simulink model "GenericTargetTemplate"  (R2022b)
settings: Solver=FixedStepAuto  StartTime=0.0  StopTime=10.0  FixedStep=0.01  RelTol=1e-3  EnableMultiTasking=on
libraries: GenericTarget x3
settings Model: Creator=damerius  LastModifiedBy=damerius
settings SolverCC: ConcurrentTasks=on  AlgebraicLoopSolver=TrustRegion  PositivePriorityOrder=on
settings DataIOCC: SaveOutput=off  SignalLogging=off  DSMLogging=off  SaveTime=off  ReturnWorkspaceOutputs=off
settings OptimizationCC: DefaultParameterBehavior=Inlined  ZeroExternalMemoryAtStartup=off  ZeroInternalMemoryAtStartup=off  SimCompilerOptimization=on
settings DebuggingCC: UnconnectedInputMsg=warning  UnconnectedOutputMsg=warning  UnconnectedLineMsg=warning  SFMachineParentedDataDiag=warning
settings HardwareCC: ProdBitPerLong=64  ProdHWDeviceType=Intel->x86-64 (Linux 64)
settings ModelReferenceCC: EnableRefExpFcnMdlSchedulingChecks=on
settings SFSimCC: SimParseCustomCode=off  SimGenImportedTypeDefs=on  SimTargetLang=C++
settings RTWCC: GenCodeOnly=on  PackageGeneratedCodeAndArtifacts=on  PackageName=PackNGo  RTWVerbose=off  BuildConfiguration=Faster Runs  TargetLang=C++  DLArmComputeVersion=19.05
settings CodeAppCC: ForceParamTrailComments=on  MaxIdLength=95  MATLABSourceComments=on  UseSimReservedNames=on
settings GRTTargetCC: TargetLangStandard=C++11 (ISO)  GenerateFullHeader=off  MatFileLogging=off  CodeInterfacePackaging=C++ class

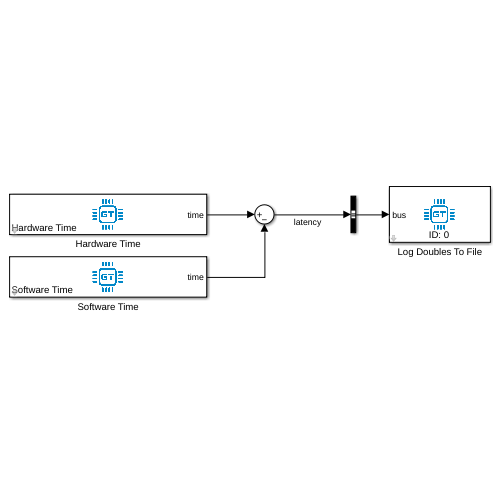
[thumbnail: Simulink's stored preview of the top-level diagram]
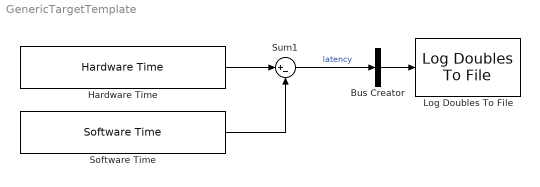
== system GenericTargetTemplate ==
  Bus Creator : BusCreator  Inputs=1
  Hardware Time : GenericTarget/Time/Hardware Time  SampleTime=0.01
      settings: SourceProductName=Generic Target
  Log Doubles To File : GenericTarget/Interface/Log Doubles To File  idLog=0  numSamplesPerFile=0  numSignals=1  signalNames=latency  numCharacters=9  SampleTime=-1
      settings: SourceProductName=Generic Target
  Software Time : GenericTarget/Time/Software Time  SampleTime=0.01
      settings: SourceProductName=Generic Target
  Sum1 : Sum  Inputs=|+-
  wires:
  Hardware Time/1 -> Sum1/1
  Software Time/1 -> Sum1/2
  Sum1/1 -> Bus Creator/1  "latency"
  Bus Creator/1 -> Log Doubles To File/1
